simulink model "SRE"  (R2021a)
settings: Solver=VariableStepAuto  StartTime=0.0  StopTime=20.0  RelTol=1e-3
values from neighbouring files (symbols this model uses):
  G = ss(Ad, Bd, Cd, Dd, Ts)    [controlador_RE.m]    (also in realim_estados_no_ff.m)
  K = acker(A_ext, B_ext, exp(Ts*p_C))    [controlador_RE.m]    (also in realim_estados_no_ff.m = [0.2533,   -0.0121, -116.5175,  -30])
  kr = inv(Cd_ff*inv(eye(4)-(Ad-Bd*K))*Bd)    [controlador_RE.m]
  L_o = [.6371, 0.0; -3.4543, 0.0; 0.0, 1.0301; -0.003, 11.1285]    [controlador_RE.m]
  Ts = 20e-3    (= 0.02)    [controlador_RE.m]    (also in realim_estados_no_ff.m)
settings Model: Creator=mathe  LastModifiedBy=mathe

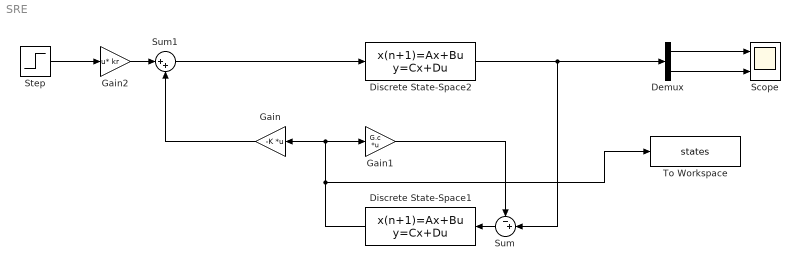
== system SRE ==
  Demux : Demux  Outputs=2
  Discrete State-Space1 : DiscreteStateSpace  A=G.a-G.b*K  B=L_o  C=eye(4)  D=zeros(4,2)  InitialCondition=[0 0 0 0]  SampleTime=Ts
  Discrete State-Space2 : DiscreteStateSpace  A=G.a  B=G.b  C=G.c  D=zeros(2,1)  InitialCondition=[0 0 0 0]  SampleTime=Ts
  Gain : Gain  Gain=-K  Multiplication=Matrix(K*u)
  Gain1 : Gain  Gain=G.c  Multiplication=Matrix(K*u)
  Gain2 : Gain  Gain=kr  Multiplication=Matrix(u*K)
  Scope : Scope  NumInputPorts=2
  Step : Step  After=0.1  SampleTime=0
  Sum : Sum  Inputs=-+|
  Sum1 : Sum  Inputs=|++
  To Workspace : ToWorkspace  VariableName=states  SampleTime=-1
      settings: Save2DSignal=2-D array (concatenate along first dimension)
  wires:
  Discrete State-Space1/1 -> To Workspace/1, Gain1/1, Gain/1
  Discrete State-Space2/1 -> Sum/2, Demux/1
  Demux/1 -> Scope/1
  Demux/2 -> Scope/2
  Sum/1 -> Discrete State-Space1/1
  Gain1/1 -> Sum/1
  Gain/1 -> Sum1/2
  Sum1/1 -> Discrete State-Space2/1
  Gain2/1 -> Sum1/1
  Step/1 -> Gain2/1
